simulink library "qqp2x"  (R2023a)
settings: Solver=VariableStepAuto  StartTime=0.0  StopTime=10.0  RelTol=1e-3
settings Model: Creator=pinki  LastModifiedBy=pinki

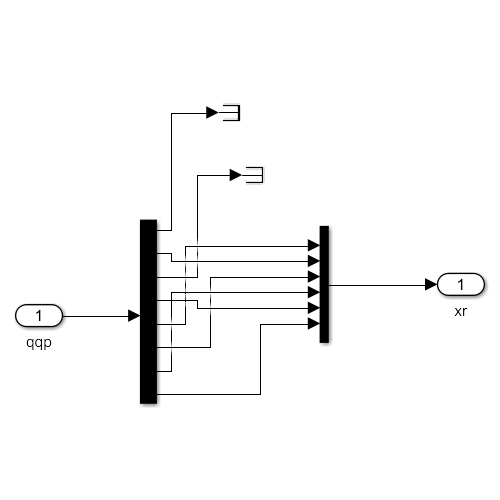
[thumbnail: Simulink's stored preview of the top-level diagram]
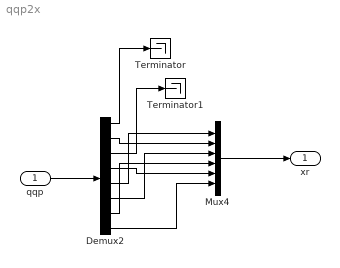
== system qqp2x ==
  qqp : Inport
  Demux2 : Demux  Outputs=8
  Mux4 : Mux  Inputs=6
  Terminator : Terminator
  Terminator1 : Terminator
  xr : Outport
  wires:
  Demux2/3 -> Terminator1/1
  qqp/1 -> Demux2/1
  Demux2/6 -> Mux4/3
  Demux2/2 -> Mux4/2
  Mux4/1 -> xr/1
  Demux2/4 -> Mux4/5
  Demux2/5 -> Mux4/1
  Demux2/7 -> Mux4/4
  Demux2/1 -> Terminator/1
  Demux2/8 -> Mux4/6
